simulink model "park_clark"  (R2024b)
settings: Solver=FixedStepAuto  StartTime=0.0  StopTime=1.0  FixedStep=1e-4  RelTol=1e-3
settings Model: Creator=86195  LastModifiedBy=86195

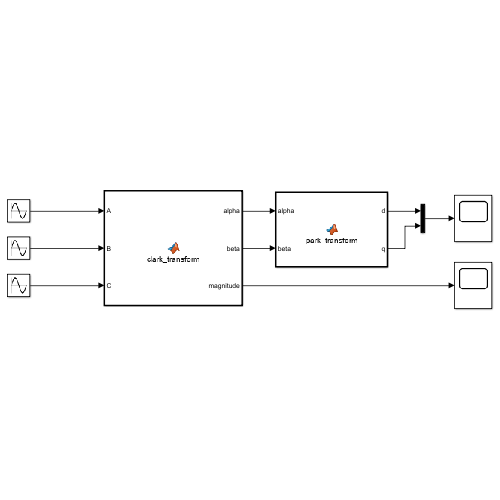
[thumbnail: Simulink's stored preview of the top-level diagram]
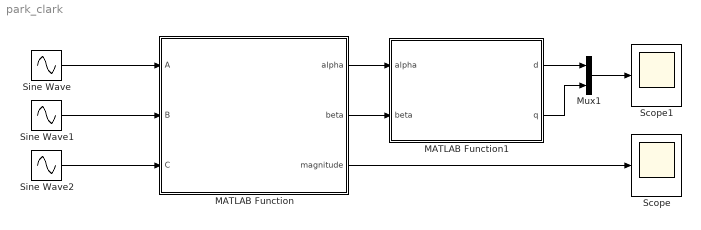
== system park_clark ==
  MATLAB Function : MATLAB Function  TreatAsAtomicUnit=on
  MATLAB Function1 : MATLAB Function  TreatAsAtomicUnit=on
  Mux1 : Mux  Inputs=2
  Scope : Scope
  Scope1 : Scope
  Sine Wave : Sin  Amplitude=220  Frequency=50*2*pi  SampleTime=0
  Sine Wave1 : Sin  Amplitude=220  Frequency=50*2*pi  Phase=120/180*pi  SampleTime=0
  Sine Wave2 : Sin  Amplitude=220  Frequency=50*2*pi  Phase=-120/180*pi  SampleTime=0
  wires:
  Sine Wave/1 -> MATLAB Function/1(A)
  Sine Wave1/1 -> MATLAB Function/2(B)
  Sine Wave2/1 -> MATLAB Function/3(C)
  MATLAB Function/3(magnitude) -> Scope/1
  MATLAB Function/1(alpha) -> MATLAB Function1/1(alpha)
  MATLAB Function/2(beta) -> MATLAB Function1/2(beta)
  MATLAB Function1/1(d) -> Mux1/1
  MATLAB Function1/2(q) -> Mux1/2
  Mux1/1 -> Scope1/1

== matlab function park_clark/MATLAB Function1 ==
  data: alpha input; d output; beta input; q output
function [d, q] = park_transform(alpha, beta)

phi = atan2(beta, alpha);
T = [cos(phi),sin(phi);
    -sin(phi), cos(phi)];
inputVector = [alpha; beta];
dqVector = T * inputVector;
d = dqVector(1);
q = dqVector(2);
end

== matlab function park_clark/MATLAB Function ==
  data: A input; alpha output; B input; C input; beta output; magnitude output
function [alpha, beta, magnitude] = clark_transform(A, B, C)
% 恒定幅值Clark变换矩阵
T = (2/3) * [1,  -1/2,      -1/2;
            0,  sqrt(3)/2, -sqrt(3)/2];
% 将三相信号转换为列向量
abc = [A; B; C];
% 应用Clark变换
alpha_beta = T * abc;
% 提取alpha和beta分量
alpha = alpha_beta(1);
beta = alpha_beta(2);
% 计算合成矢量的幅值
magnitude = sqrt(alpha^2 + beta^2);
end
